simulink model "tarea3"  (R2022b)
settings: Solver=VariableStepAuto  StartTime=0.0  StopTime=100  RelTol=1e-3
undefined symbols (not defined in the file): A, B, C, Kr_i, Kx_i, ModelMRAC, ModelReference, Ts
settings Model: Creator=felip  LastModifiedBy=felip

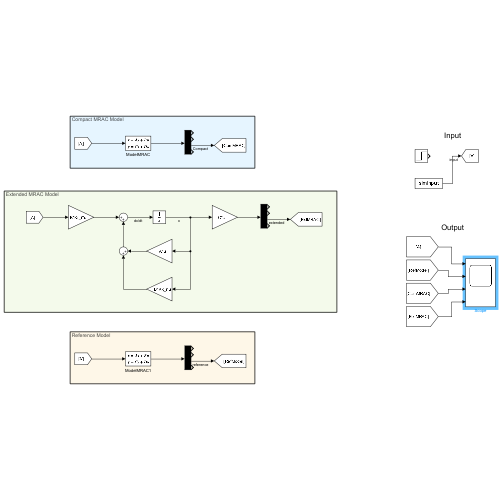
[thumbnail: Simulink's stored preview of the top-level diagram]
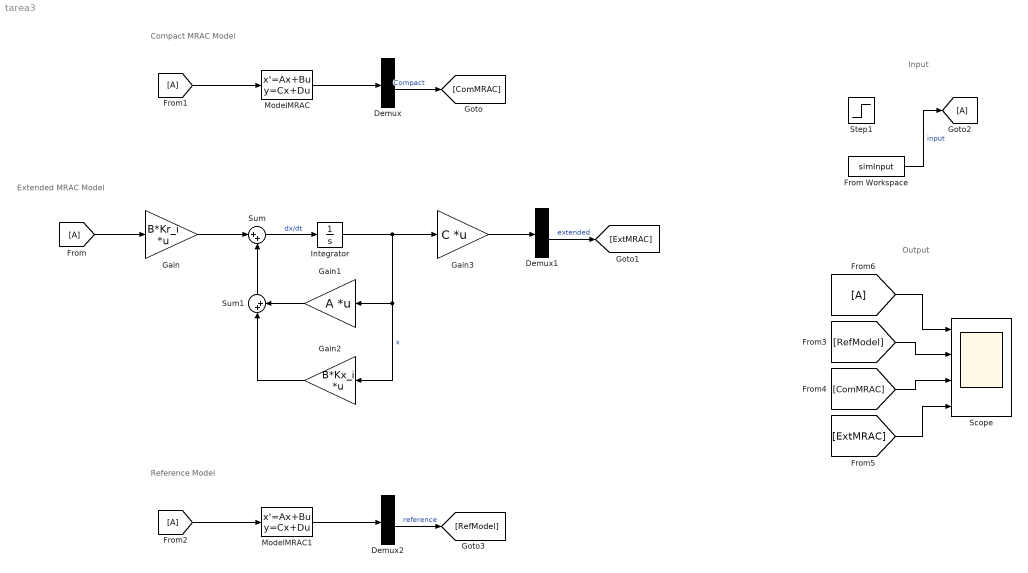
== system tarea3 ==
  note: Input
  note: Extended MRAC Model
  note: Compact MRAC Model
  note: Reference Model
  note: Output
  Demux : Demux
  Demux1 : Demux
  Demux2 : Demux
  From{,1..2,6} (4 alike) : From
  From Workspace : FromWorkspace  VariableName=simInput  SampleTime=Ts
  Gain : Gain  Gain=B*Kr_i  Multiplication=Matrix(K*u)
  Gain1 : Gain  Gain=A  Multiplication=Matrix(K*u)
  Gain2 : Gain  Gain=B*Kx_i  Multiplication=Matrix(K*u)
  Gain3 : Gain  Gain=C  Multiplication=Matrix(K*u)
  Goto2 : Goto
  Integrator : Integrator
  ModelMRAC : StateSpace  A=ModelMRAC.A  B=ModelMRAC.B  C=ModelMRAC.C  D=ModelMRAC.D  InitialCondition=0  ParameterTunability=Unconstrained
  ModelMRAC1 : StateSpace  A=ModelReference.A  B=ModelReference.B  C=ModelReference.C  D=ModelReference.D  InitialCondition=0  ParameterTunability=Unconstrained
  Scope : Scope  NumInputPorts=4
  Step1 : Step  SampleTime=0
  Sum : Sum  Inputs=|++
  Sum1 : Sum  Inputs=|++
  wires:
  From1/1 -> ModelMRAC/1
  ModelMRAC/1 -> Demux/1
  Demux/3 -> [ComMRAC]  "Compact"
  From/1 -> Gain/1
  Gain/1 -> Sum/1
  Sum/1 -> Integrator/1  "dx/dt"
  Sum1/1 -> Sum/2
  Gain1/1 -> Sum1/2
  Integrator/1 -> Gain3/1, Gain2/1, Gain1/1  "x"
  Gain2/1 -> Sum1/1
  Gain3/1 -> Demux1/1
  Demux1/3 -> [ExtMRAC]  "extended"
  From Workspace/1 -> Goto2/1  "input"
  Demux2/3 -> [RefModel]  "reference"
  From2/1 -> ModelMRAC1/1
  ModelMRAC1/1 -> Demux2/1
  [RefModel] -> Scope/2
  [ComMRAC] -> Scope/3
  [ExtMRAC] -> Scope/4
  From6/1 -> Scope/1
